simulink model "pid_model"  (R2024b)
settings: Solver=VariableStepAuto  StartTime=0.0  StopTime=10  RelTol=1e-3
values from neighbouring files (symbols this model uses):
  A = [0,1; 0,-10]    [pid_script.m]
  B = [0; 120]    [pid_script.m]
  C = [1, 0]    [pid_script.m]
  D = 0    [pid_script.m]
  Kd = 1/w_gc * dK*sin(dphi)    [pid_script.m]
  Ki = -w_gc * dK*sin(dphi)    [pid_script.m]
  Kp = dK*cos(dphi)    [pid_script.m]
  Kw = 5/ts    (= 25)    [pid_script.m]
  Tl = 1/filter_co/w_gc    (= 0.0208333333333)    [pid_script.m]
settings Model: Creator=pries  LastModifiedBy=pries

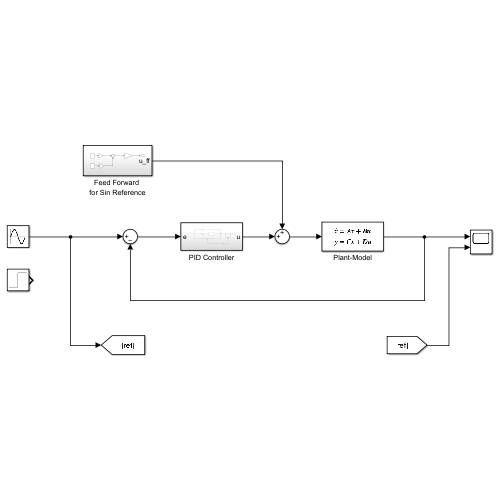
[thumbnail: Simulink's stored preview of the top-level diagram]
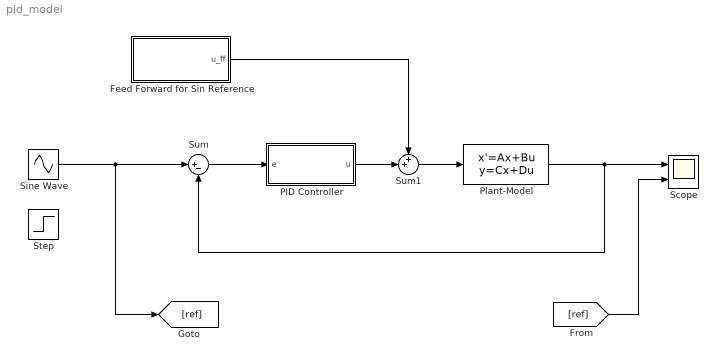
== system pid_model ==
  Feed Forward for Sin Reference : Subsystem
  PID Controller : Subsystem
  Plant-Model : StateSpace  A=A  B=B  C=C  D=D  InitialCondition=0
  Scope : Scope  NumInputPorts=2
  Sine Wave : Sin  Frequency=10  SampleTime=0
  Step : Step  Time=0  After=100  SampleTime=0
  Sum : Sum  Inputs=|+-
  Sum1 : Sum  Inputs=++|
  wires:
  Sum/1 -> PID Controller/1(e)
  Plant-Model/1 -> Scope/1, Sum/2
  PID Controller/1(u) -> Sum1/2
  Sum1/1 -> Plant-Model/1
  Feed Forward for Sin Reference/1(u_ff) -> Sum1/1
  [ref] -> Scope/2
  Sine Wave/1 -> [ref], Sum/1

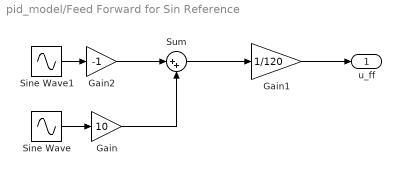
== system pid_model/Feed Forward for Sin Reference ==
  Gain : Gain  Gain=10
  Gain1 : Gain  Gain=1/120
  Gain2 : Gain  Gain=-1
  Sine Wave : Sin  Amplitude=10  Frequency=10  Phase=pi/2  SampleTime=0
  Sine Wave1 : Sin  Amplitude=100  Frequency=10  SampleTime=0
  Sum : Sum  Inputs=|++
  u_ff : Outport
  wires:
  Sine Wave1/1 -> Gain2/1
  Gain/1 -> Sum/2
  Sum/1 -> Gain1/1
  Gain1/1 -> u_ff/1
  Sine Wave/1 -> Gain/1
  Gain2/1 -> Sum/1

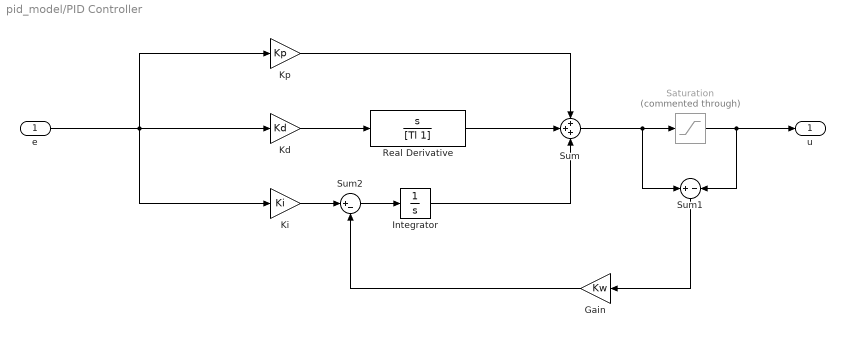
== system pid_model/PID Controller ==
  e : Inport
  Gain : Gain  Gain=Kw
  Integrator : Integrator
  Kd : Gain  Gain=Kd
  Ki : Gain  Gain=Ki
  Kp : Gain  Gain=Kp
  Real Derivative : TransferFcn  Numerator=[1,0]  Denominator=[Tl 1]
  Saturation : Saturate  Commented=through  UpperLimit=10  LowerLimit=-10
  Sum : Sum  Inputs=+++
  Sum1 : Sum  Inputs=+|-
  Sum2 : Sum  Inputs=|+-
  u : Outport
  wires:
  e/1 -> Kp/1, Ki/1, Kd/1
  Kd/1 -> Real Derivative/1
  Kp/1 -> Sum/1
  Real Derivative/1 -> Sum/2
  Integrator/1 -> Sum/3
  Sum/1 -> Sum1/1, Saturation/1
  Saturation/1 -> Sum1/2, u/1
  Sum1/1 -> Gain/1
  Gain/1 -> Sum2/2
  Ki/1 -> Sum2/1
  Sum2/1 -> Integrator/1
